simulink model "stop"  (R2021b)
settings: Solver=VariableStepAuto  StartTime=0.0  StopTime=10.0  RelTol=1e-3
libraries: dspnetwork x1
settings Model: Creator=takeh  LastModifiedBy=takeh

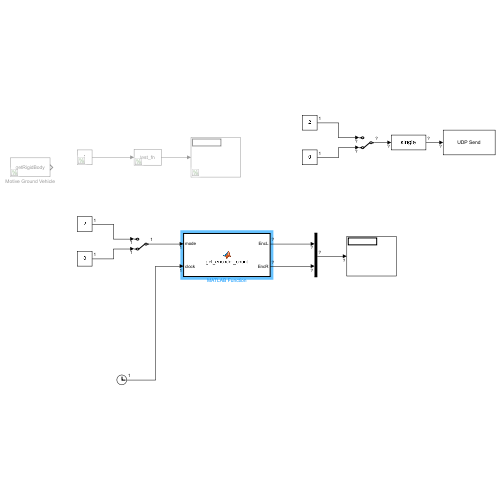
[thumbnail: Simulink's stored preview of the top-level diagram]
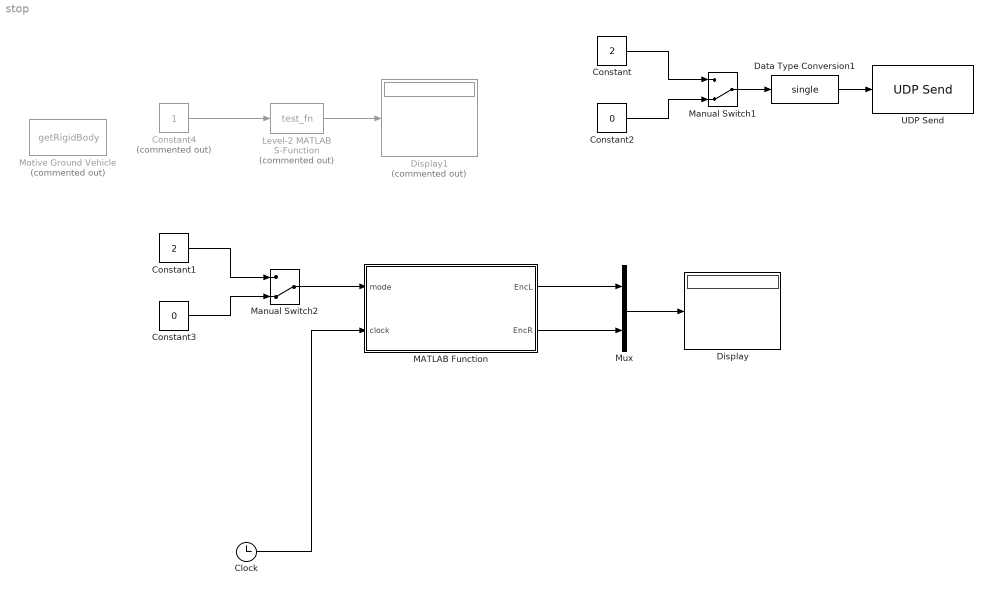
== system stop ==
  Clock : Clock
  Constant : Constant  Value=2
  Constant1 : Constant  Value=2
  Constant2 : Constant  Value=0
  Constant3 : Constant  Value=0
  Constant4 : Constant  Commented=on
  Data Type Conversion1 : DataTypeConversion  OutDataTypeStr=single
  Display : Display
  Display1 : Display  Commented=on
  Level-2 MATLAB S-Function : M-S-Function  Commented=on  FunctionName=test_fn  Parameters=1
  MATLAB Function : MATLAB Function  TreatAsAtomicUnit=on
  Manual Switch1 : ManualSwitch  CurrentSetting=0
  Manual Switch2 : ManualSwitch  CurrentSetting=0
  Motive Ground Vehicle : M-S-Function  Commented=on  FunctionName=getRigidBody  Parameters=3
  Mux : Mux  Inputs=2
  UDP Send : dspnetwork/UDP Send  remoteURL='127.0.0.1'  remotePort=52000  localURL='0.0.0.0'  localPortSource=Automatically determine  localPort=-1  sendBufferSize=8192  sampletime=-1  blockPlatform=[]  separateLengthPort=0
  wires:
  Constant2/1 -> Manual Switch1/2
  Data Type Conversion1/1 -> UDP Send/1
  Manual Switch1/1 -> Data Type Conversion1/1
  Constant/1 -> Manual Switch1/1
  Constant3/1 -> Manual Switch2/2
  Constant1/1 -> Manual Switch2/1
  Manual Switch2/1 -> MATLAB Function/1(mode)
  Clock/1 -> MATLAB Function/2(clock)
  MATLAB Function/1(EncL) -> Mux/1
  Mux/1 -> Display/1
  MATLAB Function/2(EncR) -> Mux/2
  Constant4/1 -> Level-2 MATLAB S-Function/1
  Level-2 MATLAB S-Function/1 -> Display1/1

== matlab function stop/MATLAB Function ==
  data: mode input; EncL output; clock input; EncR output
function [EncL, EncR] = get_encoder_count(mode, clock)
    Ctrl_Mode = mode;

    if clock == 0
        Port = setup;
    end

    if (Ctrl_Mode == 2)
        move;

    elseif(Ctrl_Mode == 0)
        stop;
    end
    
    if Port == None
        passthrough
    else
        [EncL, EncR] = EncoderSensorsRoomba(Port)
    end

end

function serPort = setup
    COM = 5
    Mode = 'full'
    [serPort] = RoombaInit(COM, Mode)
end

function move
    SetFwdVelRadiusRoomba(serPort, 0.1, 0)
end

function stop
    SetFwdVelRadiusRoomba(serPort, 0, 0)
end
